simulink model "lfm_characterizer"  (R2017b)
settings: Solver=VariableStepAuto  StartTime=0.0  StopTime=10.0  RelTol=1e-3
libraries: simulink x2, dspadpt3 x1, dspsnks4 x1
settings Model: Creator=rytse  LastModifiedBy=rytse

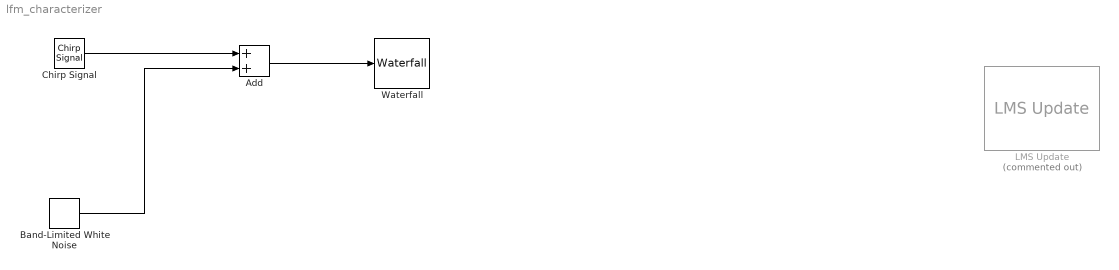
== system lfm_characterizer ==
  Add : Sum
  Band-Limited White Noise : simulink/Sources/Band-Limited White Noise  Cov=[0.1]  Ts=0.1  seed=[23341]
  Chirp Signal : simulink/Sources/Chirp Signal  f1=2e6  T=100  f2=20e6
  LMS Update : dspadpt3/LMS Update  Commented=on  Method=LMS  Length=32  StepSizeSource=Property  StepSize=0.1  LeakageFactor=1.0  InitialConditions=0  EnableAdaptInput=off  EnableResetInput=off  SimulateUsing=Code generation
      settings: SourceProductName=DSP System Toolbox  SourceProductBaseCode=DS
  Waterfall : dspsnks4/Waterfall  TraceProperties=off  NumTraces=6  CMapStr=autumn  TNewest=1  TOldest=0  HistoryLength=10  HistoryFull=Overwrite  UpdateInterval=1  ExportMode=Selected  MLExportName=ExportData  AutoExport=off  DisplayProperties=off  MouseMode=Orbit  AxisGrid=on  Snapshot=off  Suspend=off  SyncSnapshots=off  OpenScopeAtSimStart=on  FigPos=[243 195 405 320]  CameraView=[69.4600750684385 564.426060114276 -133.474523953492 0 18.5 3.5 0.616338299486424 -7.9078811427274 1.98411164834144 2.40985953613679 1 18.5 3]  InportDimsHint=[32 1]  AxisProperties=off  AxisColor='w'  XLabel=Samples  YLabel=Amplitude  ZLabel=Time  TriggerProperties=off  TrigStartMode=Immediately  TrigStartT=0  TrigStartN=0  TrigStartFcn=trigbegin  TrigStopMode=Never  TrigStopT=0.1  TrigStopN=1  TrigStopFcn=trigend  TrigRearmMode=Never  TrigRearmT=0  TrigRearmN=0  TrigRearmFcn=trigrearm  XformProperties=on  XformMode=None  XformFcn=abs  XformExpr=(u+1)/2
      settings: SourceProductName=DSP System Toolbox  SourceProductBaseCode=DS  YMin=-1  YMax=1
  wires:
  Chirp Signal/1 -> Add/1
  Band-Limited White Noise/1 -> Add/2
  Add/1 -> Waterfall/1
